simulink model "modelo_pv_testes_tamb"  (R2012b)
settings: Solver=ode45  StartTime=0.0  StopTime=10  RelTol=1e-3
values from neighbouring files (symbols this model uses):
  A = 1.3    [codigo_pv_insolacao.m]    (also in ctes_simulink_pv.m)
  Eg = 1.11    [codigo_pv_insolacao.m]    (also in ctes_simulink_pv.m)
  Isc = 3.8    [codigo_pv_insolacao.m]    (also in ctes_simulink_pv.m)
  k = 1.38e-23    [codigo_pv_insolacao.m]    (also in ctes_simulink_pv.m)
  Ki = 3e-3    (= 0.003)    [codigo_pv_insolacao.m]    (also in ctes_simulink_pv.m)
  Ns = 36    [codigo_pv_insolacao.m]    (also in ctes_simulink_pv.m)
  q = 1.6e-19    [codigo_pv_insolacao.m]    (also in ctes_simulink_pv.m)
  Tnoct = 49    [codigo_pv_insolacao.m]    (also in ctes_simulink_pv.m)
  Tref = Tref + 273    (= 298)    [codigo_pv_insolacao.m]    (also in ctes_simulink_pv.m = 25)
  Voc = 21.1    [codigo_pv_insolacao.m]    (also in ctes_simulink_pv.m)
settings Model: Creator=Eduardo Raguenet  LastModifiedBy=Eduardo Raguenet

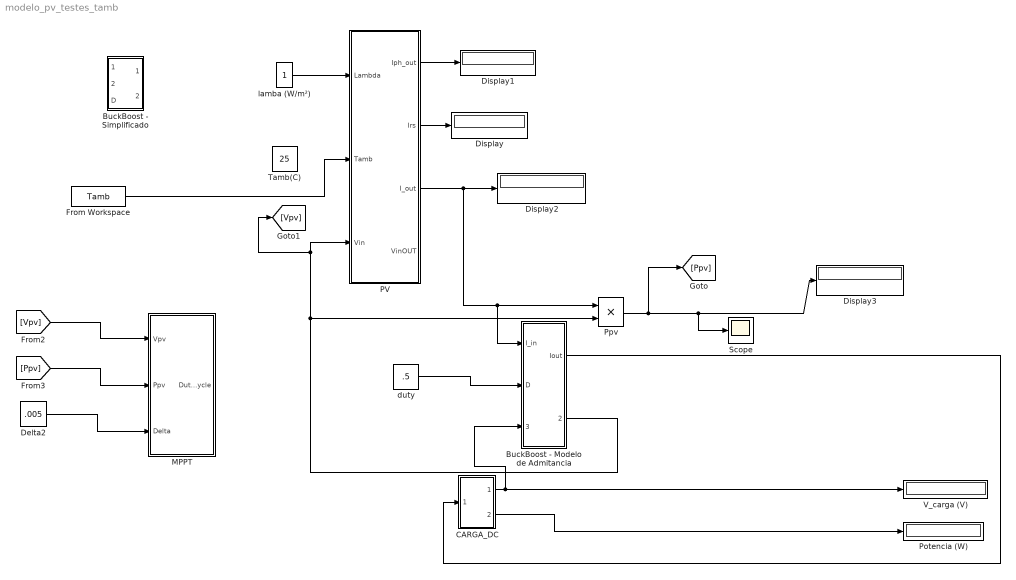
== system modelo_pv_testes_tamb ==
  BuckBoost - Modelo de Admitancia : Subsystem
  BuckBoost - Simplificado : Subsystem
  CARGA_DC : Subsystem
  Delta2 : Constant  Value=.005
  Display{,1..3} (4 alike) : Display
  From Workspace : FromWorkspace  VariableName=Tamb  SampleTime=0
  MPPT : Subsystem
  PV : Subsystem
  Potencia (W) : Display
  Ppv : Product  Inputs=**
  Scope : Scope
      settings: YMin=0  YMax=8.5e-16
  "Tamb(C) " : Constant  Value=25
  V_carga (V) : Display
  duty : Constant  Value=.5
  lamba (W/m²) : Constant
  wires:
  PV/1(Iph_out) -> Display1/1
  lamba (W/m²)/1 -> PV/1("Lambda ")
  PV/2(Irs) -> Display/1
  PV/3(I_out) -> BuckBoost - Modelo de Admitancia/1(I_in), Ppv/1, Display2/1
  CARGA_DC/2(P_carga) -> Potencia (W)/1
  Ppv/1 -> [Ppv], Scope/1, Display3/1
  BuckBoost - Modelo de Admitancia/1(Iout) -> CARGA_DC/1(I_carga)
  CARGA_DC/1(V_carga) -> V_carga (V)/1, BuckBoost - Modelo de Admitancia/3(Vout_carga)
  BuckBoost - Modelo de Admitancia/2(Vin_PV) -> Ppv/2, [Vpv], PV/3(Vin)
  [Vpv] -> MPPT/1(Vpv)
  [Ppv] -> MPPT/2(Ppv)
  Delta2/1 -> MPPT/3(Delta)
  duty/1 -> BuckBoost - Modelo de Admitancia/2(D)
  From Workspace/1 -> PV/2(Tamb)

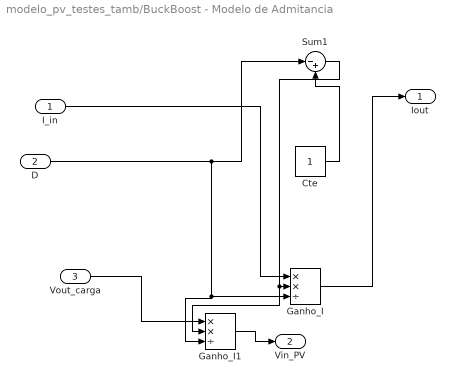
== system modelo_pv_testes_tamb/BuckBoost - Modelo de Admitancia ==
  I_in : Inport
  D : Inport  Port=2
  Vout_carga : Inport  Port=3
  Cte : Constant
  Ganho_I : Product  Inputs=**/
  Ganho_I1 : Product  Inputs=**/
  Sum1 : Sum  Inputs=|-+
  Iout : Outport
  Vin_PV : Outport  Port=2
  wires:
  Cte/1 -> Sum1/2
  I_in/1 -> Ganho_I/1
  Ganho_I/1 -> Iout/1
  Sum1/1 -> Ganho_I1/2, Ganho_I/2
  D/1 -> Ganho_I1/3, Ganho_I/3, Sum1/1
  Vout_carga/1 -> Ganho_I1/1
  Ganho_I1/1 -> Vin_PV/1

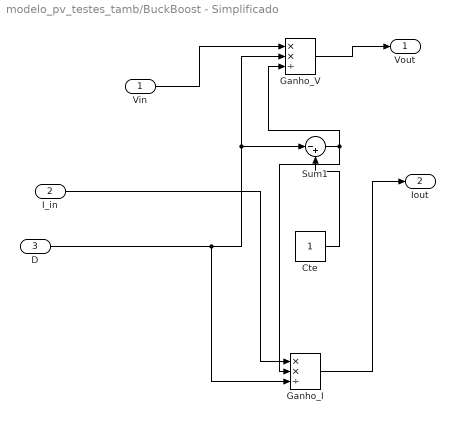
== system modelo_pv_testes_tamb/BuckBoost - Simplificado ==
  Vin : Inport
  I_in : Inport  Port=2
  D : Inport  Port=3
  Cte : Constant
  Ganho_I : Product  Inputs=**/
  Ganho_V : Product  Inputs=**/
  Sum1 : Sum  Inputs=|-+
  Vout : Outport
  Iout : Outport  Port=2
  wires:
  Cte/1 -> Sum1/2
  I_in/1 -> Ganho_I/1
  Ganho_I/1 -> Iout/1
  Sum1/1 -> Ganho_I/2, Ganho_V/3
  D/1 -> Ganho_I/3, Sum1/1, Ganho_V/2
  Vin/1 -> Ganho_V/1
  Ganho_V/1 -> Vout/1

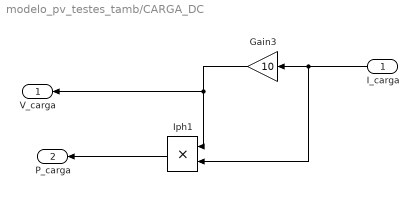
== system modelo_pv_testes_tamb/CARGA_DC ==
  I_carga : Inport
  Gain3 : Gain  Gain=10
  Iph1 : Product  Inputs=**
  V_carga : Outport
  P_carga : Outport  Port=2
  wires:
  Iph1/1 -> P_carga/1
  Gain3/1 -> V_carga/1, Iph1/1
  I_carga/1 -> Iph1/2, Gain3/1

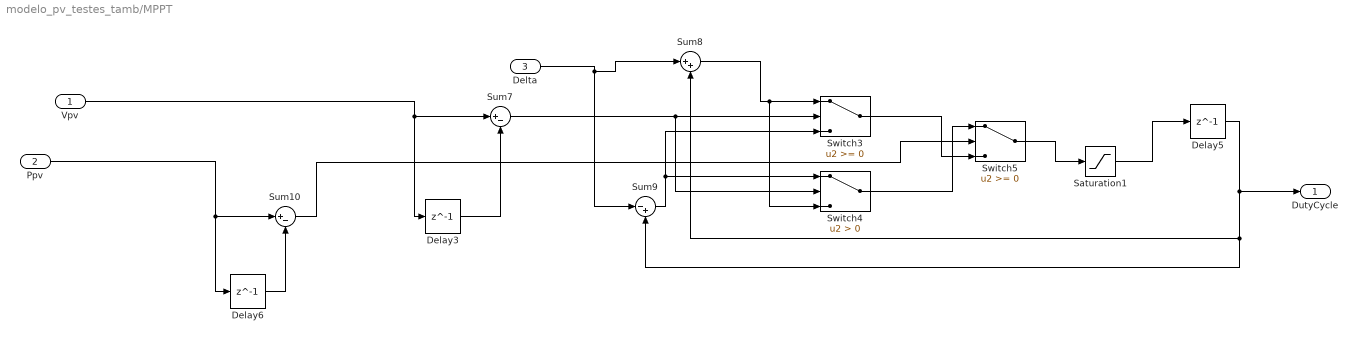
== system modelo_pv_testes_tamb/MPPT ==
  Vpv : Inport
  Ppv : Inport  Port=2
  Delta : Inport  Port=3
  Delay3 : Delay  DelayLength=1  InitialCondition=0  SampleTime=1e-2
  Delay5 : Delay  DelayLength=1  InitialCondition=.5  SampleTime=1e-2
  Delay6 : Delay  DelayLength=1  InitialCondition=0  SampleTime=1e-2
  Saturation1 : Saturate  UpperLimit=1  LowerLimit=0
  Sum10 : Sum  Inputs=|+-
  Sum7 : Sum  Inputs=|+-
  Sum8 : Sum  Inputs=|++
  Sum9 : Sum  Inputs=|-+
  Switch3 : Switch
  Switch4 : Switch  Criteria=u2 > Threshold
  Switch5 : Switch
  DutyCycle : Outport
  wires:
  Sum7/1 -> Switch4/2, Switch3/2
  Switch4/1 -> Switch5/1
  Switch3/1 -> Switch5/3
  Delay3/1 -> Sum7/2
  Delay5/1 -> DutyCycle/1, Sum9/2, Sum8/2
  Switch5/1 -> Saturation1/1
  Saturation1/1 -> Delay5/1
  Sum8/1 -> Switch4/3, Switch3/1
  Sum9/1 -> Switch4/1, Switch3/3
  Vpv/1 -> Delay3/1, Sum7/1
  Sum10/1 -> Switch5/2
  Ppv/1 -> Delay6/1, Sum10/1
  Delay6/1 -> Sum10/2
  Delta/1 -> Sum9/1, Sum8/1

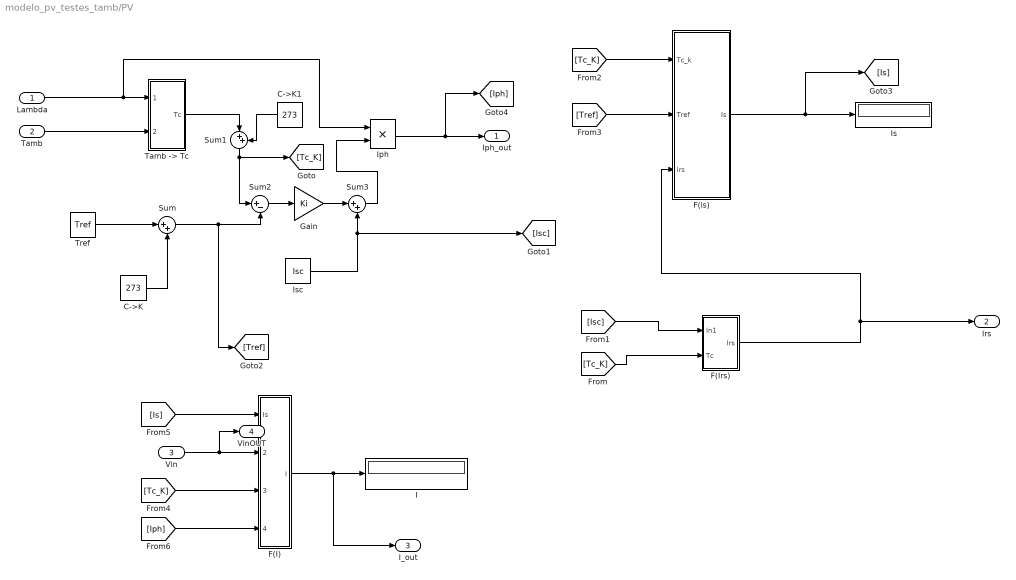
== system modelo_pv_testes_tamb/PV ==
  "Lambda " : Inport
  Tamb : Inport  Port=2
  Vin : Inport  Port=3
  C->K : Constant  Value=273
  C->K1 : Constant  Value=273
  F(I) : Subsystem
  F(Irs) : Subsystem
  F(is) : Subsystem
  Gain : Gain  Gain=Ki
  I : Display
  Iph : Product  Inputs=**
  Is : Display
  Isc : Constant  Value=Isc
  Sum : Sum  Inputs=|++
  Sum1 : Sum  Inputs=|++
  Sum2 : Sum  Inputs=|+-
  Sum3 : Sum  Inputs=|++
  "Tamb -> Tc" : Subsystem
  Tref : Constant  Value=Tref
  Iph_out : Outport
  Irs : Outport  Port=2
  I_out : Outport  Port=3
  VinOUT : Outport  Port=4
  wires:
  Sum3/1 -> Iph/2
  "Tamb -> Tc"/1(Tc) -> Sum1/1
  C->K1/1 -> Sum1/2
  Sum2/1 -> Gain/1
  Tref/1 -> Sum/1
  C->K/1 -> Sum/2
  Tamb/1 -> "Tamb -> Tc"/2(Tamb)
  "Lambda "/1 -> Iph/1, "Tamb -> Tc"/1(Lambda)
  Gain/1 -> Sum3/1
  Isc/1 -> Sum3/2, [Isc]
  Sum/1 -> [Tref], Sum2/2
  Sum1/1 -> Sum2/1, [Tc_K]
  Iph/1 -> [Iph], Iph_out/1
  F(Irs)/1(Irs) -> Irs/1, F(is)/3(Irs)
  [Isc] -> F(Irs)/1(In1)
  [Tc_K] -> F(Irs)/2(Tc)
  [Tc_K] -> F(is)/1(Tc_k)
  [Tref] -> F(is)/2(Tref)
  F(is)/1(Is) -> [Is], Is/1
  [Is] -> F(I)/1(Is)
  Vin/1 -> VinOUT/1, F(I)/2(Vin)
  [Tc_K] -> F(I)/3(TC_K)
  [Iph] -> F(I)/4(Iph)
  F(I)/1(I) -> I_out/1, I/1

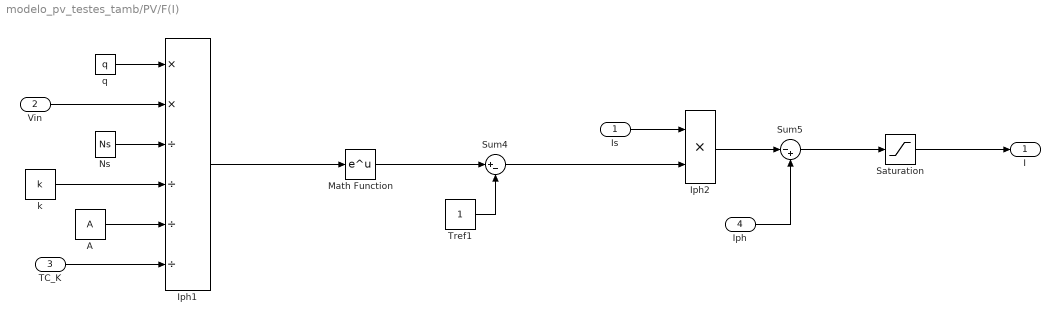
== system modelo_pv_testes_tamb/PV/F(I) ==
  Is : Inport
  Vin : Inport  Port=2
  TC_K : Inport  Port=3
  Iph : Inport  Port=4
  A : Constant  Value=A
  Iph1 : Product  Inputs=**////
  Iph2 : Product  Inputs=**
  Math Function : Math  OutputSignalType=real  SaturateOnIntegerOverflow=on
  Ns : Constant  Value=Ns
  Saturation : Saturate  UpperLimit=100  LowerLimit=0
  Sum4 : Sum  Inputs=|+-
  Sum5 : Sum  Inputs=|-+
  Tref1 : Constant
  k : Constant  Value=k
  q : Constant  Value=q
  I : Outport
  wires:
  TC_K/1 -> Iph1/6
  q/1 -> Iph1/1
  k/1 -> Iph1/4
  Is/1 -> Iph2/1
  Iph/1 -> Sum5/2
  Iph2/1 -> Sum5/1
  Math Function/1 -> Sum4/1
  A/1 -> Iph1/5
  Ns/1 -> Iph1/3
  Tref1/1 -> Sum4/2
  Vin/1 -> Iph1/2
  Iph1/1 -> Math Function/1
  Sum4/1 -> Iph2/2
  Sum5/1 -> Saturation/1
  Saturation/1 -> I/1

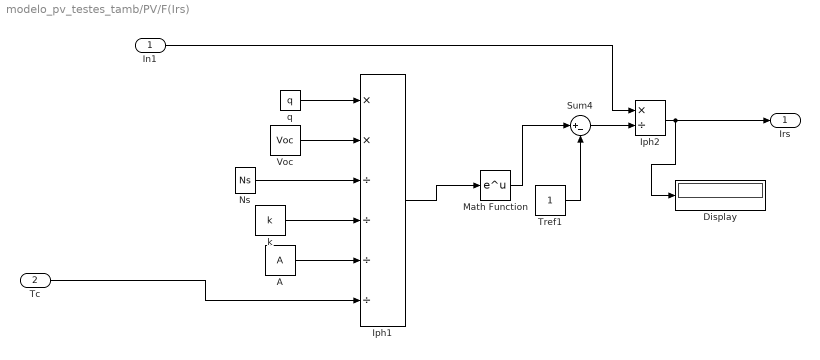
== system modelo_pv_testes_tamb/PV/F(Irs) ==
  In1 : Inport
  Tc : Inport  Port=2
  A : Constant  Value=A
  Display : Display
  Iph1 : Product  Inputs=**////
  Iph2 : Product  Inputs=*/
  Math Function : Math  OutputSignalType=real  SaturateOnIntegerOverflow=on
  Ns : Constant  Value=Ns
  Sum4 : Sum  Inputs=|+-
  Tref1 : Constant
  Voc : Constant  Value=Voc
  k : Constant  Value=k
  q : Constant  Value=q
  Irs : Outport
  wires:
  Ns/1 -> Iph1/3
  Tref1/1 -> Sum4/2
  Tc/1 -> Iph1/6
  Sum4/1 -> Iph2/2
  k/1 -> Iph1/4
  A/1 -> Iph1/5
  Math Function/1 -> Sum4/1
  q/1 -> Iph1/1
  In1/1 -> Iph2/1
  Voc/1 -> Iph1/2
  Iph2/1 -> Irs/1, Display/1
  Iph1/1 -> Math Function/1

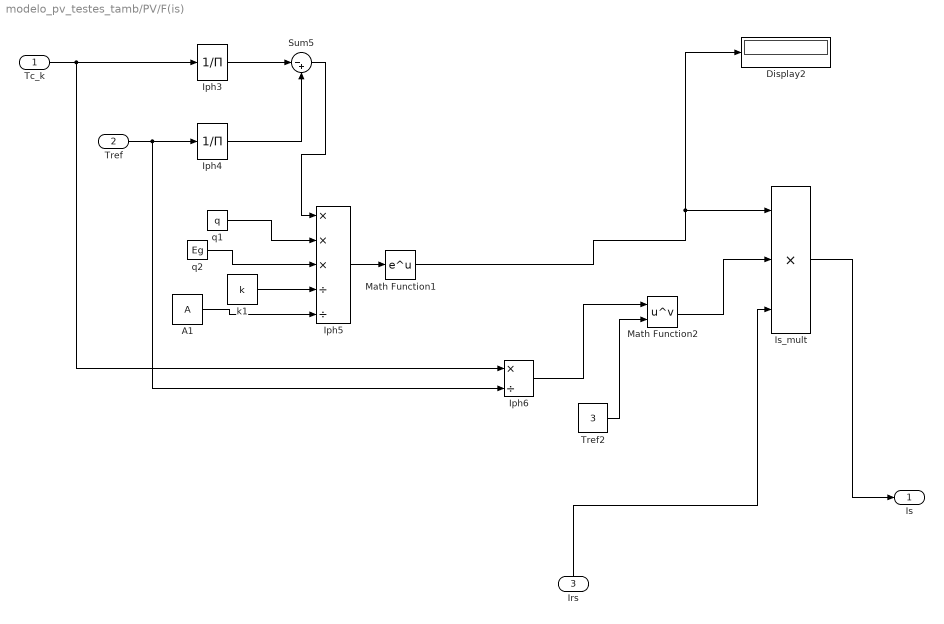
== system modelo_pv_testes_tamb/PV/F(is) ==
  Tc_k : Inport
  Tref : Inport  Port=2
  Irs : Inport  Port=3
  A1 : Constant  Value=A
  Display2 : Display
  Iph3 : Product  Inputs=/
  Iph4 : Product  Inputs=/
  Iph5 : Product  Inputs=***//
  Iph6 : Product  Inputs=*/
  Is_mult : Product  Inputs=***
  Math Function1 : Math  OutputSignalType=real  SaturateOnIntegerOverflow=on
  Math Function2 : Math  Operator=pow  OutputSignalType=real  SaturateOnIntegerOverflow=on
  Sum5 : Sum  Inputs=|-+
  Tref2 : Constant  Value=3
  k1 : Constant  Value=k
  q1 : Constant  Value=q
  q2 : Constant  Value=Eg
  Is : Outport
  wires:
  Iph5/1 -> Math Function1/1
  Irs/1 -> Is_mult/3
  Tref/1 -> Iph6/2, Iph4/1
  Iph3/1 -> Sum5/1
  Tref2/1 -> Math Function2/2
  Iph6/1 -> Math Function2/1
  Sum5/1 -> Iph5/1
  Tc_k/1 -> Iph6/1, Iph3/1
  Is_mult/1 -> Is/1
  Math Function2/1 -> Is_mult/2
  k1/1 -> Iph5/4
  q1/1 -> Iph5/2
  A1/1 -> Iph5/5
  Iph4/1 -> Sum5/2
  Math Function1/1 -> Is_mult/1, Display2/1
  q2/1 -> Iph5/3

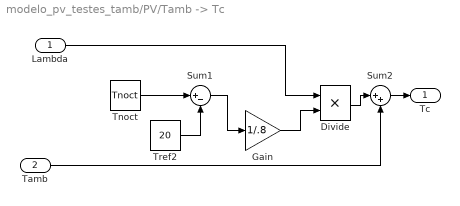
== system modelo_pv_testes_tamb/PV/Tamb -> Tc ==
  Lambda : Inport
  Tamb : Inport  Port=2
  Divide : Product  Inputs=**
  Gain : Gain  Gain=1/.8
  Sum1 : Sum  Inputs=|+-
  Sum2 : Sum  Inputs=|++
  Tnoct : Constant  Value=Tnoct
  Tref2 : Constant  Value=20
  Tc : Outport
  wires:
  Tnoct/1 -> Sum1/1
  Tamb/1 -> Sum2/2
  Tref2/1 -> Sum1/2
  Lambda/1 -> Divide/1
  Sum2/1 -> Tc/1
  Divide/1 -> Sum2/1
  Sum1/1 -> Gain/1
  Gain/1 -> Divide/2
